simulink model "Acc_Interface"  (R2024b)
settings: Solver=FixedStepAuto  StartTime=0.0  StopTime=inf  FixedStep=1e-3  RelTol=1e-3
InitFcn:
  | run('config.m');
libraries: arduinolib x2
settings Model: ExtModeTrigDuration=2  Creator=Marc  LastModifiedBy=Nitesh
settings SolverCC: AutoInsertRateTranBlk=on
settings OptimizationCC: DefaultParameterBehavior=Inlined  GainParamInheritBuiltInType=on  UseFloatMulNetSlope=on  InlineInvariantSignals=on  EnhancedBackFolding=on  PassReuseOutputArgsAs=Individual arguments  ZeroExternalMemoryAtStartup=off  ZeroInternalMemoryAtStartup=off  EfficientFloat2IntCast=on  MaxStackSize=64  OptimizeBlockOrder=speed  DifferentSizesBufferReuse=on  OptimizationCustomize=off  EfficientTunableParamExpr=on
settings DebuggingCC: SaveWithParameterizedLinksMsg=none  UnderspecifiedInitializationDetection=Classic  MergeDetectMultiDrivingBlocksExec=none  SignalResolutionControl=TryResolveAllWithWarning  ParameterTunabilityLossMsg=error
settings HardwareCC: ProdBitPerPointer=32  ProdBitPerSizeT=32  ProdBitPerPtrDiffT=32  ProdLargestAtomicInteger=Long  ProdLargestAtomicFloat=Double  ProdWordSize=32  ProdHWDeviceType=ARM Compatible->ARM Cortex  TargetIntDivRoundTo=Zero  TargetEndianess=LittleEndian  TargetHWDeviceType=Custom Processor->Custom Processor  ProdEqTarget=off  UseEmbeddedCoderFeatures=off
settings ModelReferenceCC: PropagateSignalLabelsOutOfModel=off
settings RTWCC: Description=Embedded Coder  SystemTargetFile=ert.tlc  HardwareBoard=ESP32-WROOM(Arduino Compatible)  TLCOptions="-aInlineSetEventsForThisBaseRateFcn=TLC_FALSE -aSuppressMultiTaskScheduler=TLC_FALSE  -aRateBasedStepFcn=0"  TemplateMakefile=ert_default_tmf  Toolchain=ESP32  BuildConfiguration=Faster Runs
settings CodeAppCC: ForceParamTrailComments=on  IgnoreCustomStorageClasses=off  OperatorAnnotations=on  SimulinkDataObjDesc=on  SFDataObjDesc=on  InsertBlockDesc=on
settings ERTTargetCC: SupportNonFinite=off  SupportContinuousTime=on  SupportNonInlinedSFcns=on  SupportVariableSizeSignals=on  ExtModeTransport=3  ExtModeStaticAlloc=on  ExtModeAutomaticAllocSize=off  ExtModeStaticAllocSize=65536  ExtModeMexFile=ext_xcp  ExtModeIntrfLevel=Level2 - Open  InlinedParameterPlacement=Hierarchical

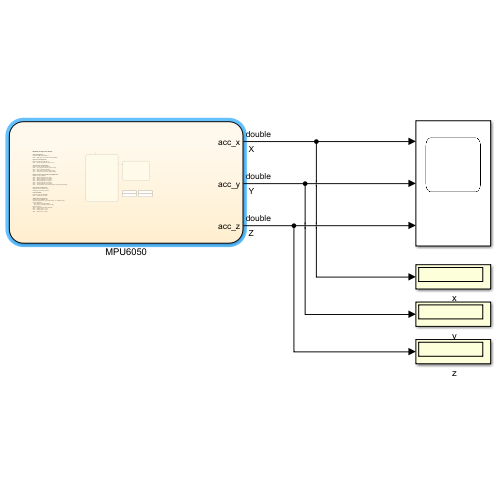
[thumbnail: Simulink's stored preview of the top-level diagram]
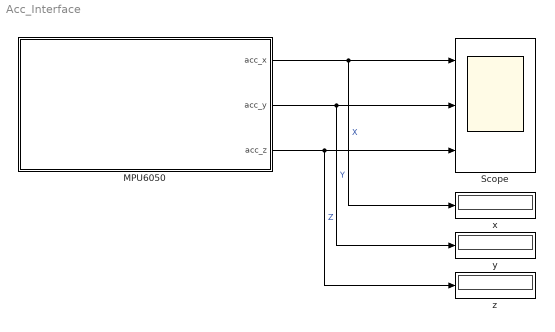
== system Acc_Interface ==
  " x" : Display
  " y" : Display
  " z" : Display
  MPU6050 : Stateflow chart  TreatAsAtomicUnit=on
      settings: PortSchema="{\"entries\":[{\"content\":{\"sides\":[{\"content\":{},\"type\":\"ConnectorPlacement.EquallySpacedRectSide\",\"uuid\":\"e0cad0cf-2ed8-4cf7-bff6-6ed2feffa650\"},{\"content\":{\"connectorIds\":[\"Out1\",\"Out3\",\"Out2\"],\"side\":\"RIGHT\"},\"type\":\"ConnectorPlacement.EquallySpacedRectSide\",\"uuid\":\"9c27c799-2435-4d39-8ba1-4c3814f68cde\"},{\"content\":{\"side\":\"TOP\"},\"type\":\"ConnectorPlacement.EquallySpacedRectSide\",\"uuid\":\"52d11aab-2c42-4a19-9ee0-cf61f3e3e234\"}]},\"type\":\"ConnectorPlacement.EquallySpacedConnector\",\"uuid\":\"b37ebc91-bb9d-4b35-9b01-6a26108d89d3\"}],\"packageUris\":[\"http://schema.mathworks.com/mf0/Connector/R2020b\"],\"version\":\"1.0\"}"
  Scope : Scope  NumInputPorts=3
  wires:
  MPU6050/1(acc_x) -> " x"/1, Scope/1  "X"
  MPU6050/3(acc_y) -> " y"/1, Scope/2  "Y"
  MPU6050/2(acc_z) -> " z"/1, Scope/3  "Z"

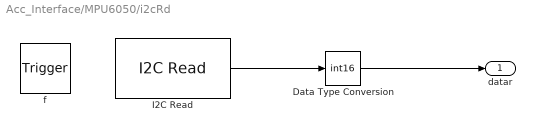
== system Acc_Interface/MPU6050/i2cRd ==
  f : TriggerPort  TriggerType=function-call  VariantControl=Variant  SampleTime=inf
      settings: CopyFcn=Stateflow.SLINSF.SimulinkMan.removeBlockPreDeleteFcn  PreDeleteFcn=Stateflow.SLINSF.SimulinkMan.unsafePredeleteFcn
  Data Type Conversion : DataTypeConversion  OutDataTypeStr=int16  SaturateOnIntegerOverflow=off  RndMeth=Floor
  I2C Read : arduinolib/I2C Read  I2CModule=0  Mode=Master  SlaveAddress=hex2dec( '68' )  SlaveByteOrder=BigEndian  Direction=Receiver  RegisterAddressMode=on  RegisterAddress=hex2dec( '3b' )  SlaveDataType=uint16  DataLength=3  NoAck=off  RepeatedStart=off  OutputStatus=off  blockPlatform=arduino  SampleTime=-1
      settings: SourceProductName=Common
  datar : Outport  Unit=1  VectorParamsAs1DForOutWhenUnconnected=off
  wires:
  I2C Read/1 -> Data Type Conversion/1
  Data Type Conversion/1 -> datar/1

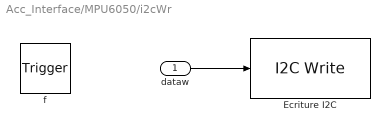
== system Acc_Interface/MPU6050/i2cWr ==
  dataw : Inport  OutDataTypeStr=uint16  Unit=1  PortDimensions=1
  f : TriggerPort  TriggerType=function-call  VariantControl=Variant  SampleTime=-1
      settings: CopyFcn=Stateflow.SLINSF.SimulinkMan.removeBlockPreDeleteFcn  PreDeleteFcn=Stateflow.SLINSF.SimulinkMan.unsafePredeleteFcn
  Ecriture I2C : arduinolib/I2C Write  Priority=1  I2CModule=0  Mode=Master  SlaveAddress=hex2dec( '68' )  SlaveByteOrder=BigEndian  Direction=Transmitter  RegisterAddressMode=off  RegisterAddress=hex2dec( '6B' )  SlaveDataType=uint16  DataLength=1  NoAck=off  RepeatedStart=off  OutputStatus=off  blockPlatform=arduino
      settings: SourceProductName=Common
  wires:
  dataw/1 -> Ecriture I2C/1

== stateflow chart Acc_Interface/MPU6050 ==
  note: MPU6050 Configuration Details
      |
      | Power Management :
      | Register: 0x6B (PWR_MGMT_1)
      | 0x00 → Wake up & use internal oscillator (8MHz)
      |
      | Gyroscope Configuration:
      | Register: 0x6C (PWR_MGMT_2)
      | 0x07 → Disable all gyroscope axes (X, Y, Z)
      |
      | Accelerometer Configuration :
      | Register: 0x1C (ACCEL_CONFIG)
      | 0x00 → ±2g (highest sensitivity, lowest range)
      | 0x08 → ±4g (moderate sensitivity)
      | 0x10 → ±8g (lower sensitivity, higher range)
      | 0x18 → ±16g (lowest sensitivity, highest range)
      |
      | Digital Low-Pass Filter (DLPF) and Update Rate:
      | Register: 0x1A (CONFIG)
      | 0x00 → 260Hz bandwidth, 0ms delay
      | 0x01 → 184Hz bandwidth, 2.0ms delay
      | 0x02 → 94Hz bandwidth, 3.0ms delay
      | 0x03 → 44Hz bandwidth, 4.9ms delay
      | 0x04 → 21Hz bandwidth, 8.5ms delay
      | 0x05 → 10Hz bandwidth, 13.8ms delay
      | 0x06 → 5Hz bandwidth, 19.0ms delay (lowest noise, highest filtering)
      |
      | Interrupt Pin Configuration:
      | Register: 0x37 (INT_PIN_CFG)
      | Configures interrupt pin behavior
      |
      | Interrupt Enable:
      | Register: 0x38 (INT_ENABLE)
      | 0x00 → Disable all interrupts
      |
      | Sample Rate Configuration:
      | Register: 0x19 (SMPLRT_DIV)
      | Formula: Sample Rate = Gyro Output Rate / (1 + SMPLRT_DIV)
      | Gyro Output Rate:
      | - 8kHz if DLPF is disabled (0x00)
      | - 1kHz if DLPF is enabled (0x01 to 0x06)
      | Example values:
      | 0x00 → 1kHz (default if DLPF enabled)
      | 0x07 → 125Hz (1kHz / (1+7))
      | 0x13 → 50Hz (1kHz / (1+19))
      | 0x27 → 25Hz (1kHz / (1+39))
  note: initialisation
      | en:
      | % -------------- Power Management --------------
      | i2cWr(uint16(hex2dec('6B00'))); % Power on
      | % Check if Gyroscope should be disabled
      | if ~ENABLE_GYRO
      |     i2cWr(uint16(hex2dec('6C07'))); % Disable Gyroscope
      | else
      |     i2cWr(uint16(hex2dec('6C00'))); % Enable Gyroscope
      | end
      | % -------------- Accelerometer Configuration --------------
      | switch ACCEL_RANGE
      |     case uint8(2)
      |         i2cWr(uint16(0x1C00));
      |         scale_factor = 16384;  % ±2g
      |     case uint8(4)
      |         i2cWr(uint16(0x1C08));
      |         scale_factor = 8192;   % ±4g
      |     case uint8(8)
      |         i2cWr(uint16(0x1C10));
      |         scale_factor = 4096;   % ±8g
      |     case uint8(16)
      |         i2cWr(uint16(0x1C18));
      |         scale_factor = 2048;   % ±16g
      |     otherwise
      |         error('Invalid Accelerometer Range');
      | end
      | % -------------- Digital Low-Pass Filter --------------
      | if DLPF_SETTING >= 0 && DLPF_SETTING <= 6
      |     i2cWr(uint16(0x1A00) + uint16(DLPF_SETTING));
      | else
      |     error('Invalid DLPF setting');
      | end
      | % -------------- Sampling Configuration --------------
      | % Ensure SAMPLE_RATE_DIV is uint8
      | i2cWr(bitor(0x1900, uint16(uint8(SAMPLE_RATE_DIV))));
      | % -------------- Interrupts --------------
      | i2cWr(uint16(hex2dec('3710'))); % Interrupt pin setup
      | i2cWr(uint16(hex2dec('3800'))); % Disable interrupts
      | disp('MPU6050 Initialization Completed.');
  state initialisation
    en:
    % -------------- Power Management --------------
    i2cWr(uint16(hex2dec('6B00'))); % Power on
    % Check if Gyroscope should be disabled
    if ~ENABLE_GYRO
    i2cWr(uint16(hex2dec('6C07'))); % Disable Gyroscope
    else
    i2cWr(uint16(hex2dec('6C00'))); % Enable Gyroscope
    end
    % -------------- Accelerometer Configuration --------------
    switch ACCEL_RANGE
    case uint8(2)
    i2cWr(uint16(0x1C00));
    scale_factor = 16384;  % ±2g
    case uint8(4)
    i2cWr(uint16(0x1C08));
    scale_factor = 8192;   % ±4g
    case uint8(8)
    i2cWr(uint16(0x1C10));
    scale_factor = 4096;   % ±8g
    case uint8(16)
    i2cWr(uint16(0x1C18));
    scale_factor = 2048;   % ±16g
    otherwise
    error('Invalid Accelerometer Range');
    end
    % -------------- Digital Low-Pass Filter --------------
    if DLPF_SETTING >= 0 && DLPF_SETTING <= 6
    i2cWr(uint16(0x1A00) + uint16(DLPF_SETTING));
    else
    error('Invalid DLPF setting');
    end
    disp('MPU6050 Initialization Completed.');
  state MPU_Running
    during:
    % Read raw data from MPU6050
    val = i2cRd;
    % Extract acceleration values (X, Y, Z)
    raw_acc_x=val(1);
    raw_acc_y=val(2);
    raw_acc_z=val(3);
    %
    acc_x = double(raw_acc_x) / double(scale_factor);
    acc_y = double(raw_acc_y) / double(scale_factor);
    acc_z = double(raw_acc_z) / double(scale_factor);
  state i2cWr(dataw) [function]
  state datar = i2cRd [function]
  (default) -> initialisation
  initialisation -> MPU_Running
  data: dataw function_input uint16 size=1; datar function_output; val local int16 size=3; acc_x output double; acc_z output double; acc_y output double; raw_acc_x local int16; raw_acc_y local int16; raw_acc_z local int16; scale_factor local uint16 =1; ENABLE_GYRO constant double; ACCEL_RANGE parameter uint8; SAMPLE_RATE_DIV constant double; DLPF_SETTING constant double; scale_factors local; accel_cmds local
